simulink library "SG_send_servo_valve_position_command"  (R2025b)
settings: Solver=VariableStepAuto  StartTime=0.0  StopTime=10.0  RelTol=1e-3
libraries: simulink x2, slrealtimeseriallib x2, hdlsllib x1
settings Model: Creator=cmmcguir  LastModifiedBy=cmmcguir

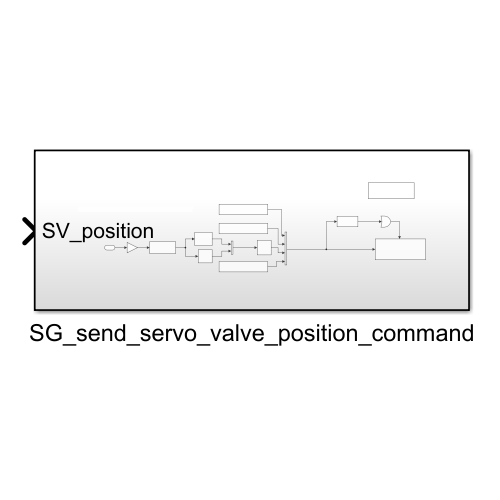
[thumbnail: Simulink's stored preview of the top-level diagram]
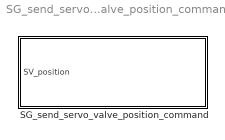
== system SG_send_servo_valve_position_command ==
  SG_send_servo_valve_position_command : Subsystem

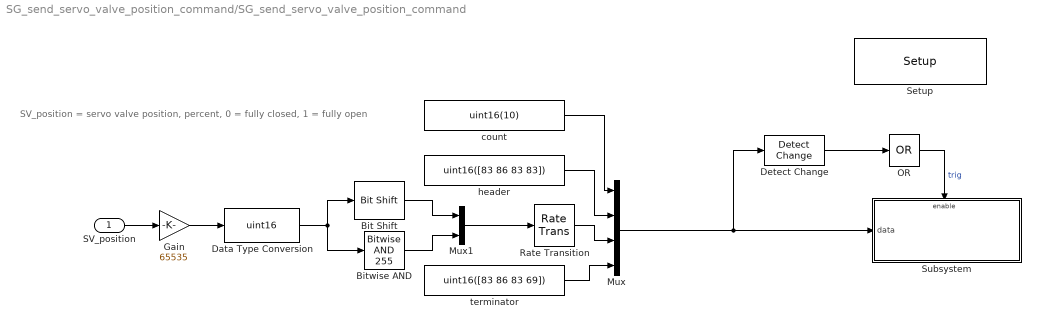
== system SG_send_servo_valve_position_command/SG_send_servo_valve_position_command ==
  note: SV_position = servo valve position, percent, 0 = fully closed, 1 = fully open
  SV_position : Inport
  Bit Shift : hdlsllib/Logic and Bit Operations/Bit Shift  mode=Shift Right Logical  N=8
  Bitwise AND : simulink/Logic and Bit Operations/Bitwise Operator  logicop=AND  UseBitMask=on  BitMask=255  BitMaskRealWorld=Stored Integer
      settings: LibrarySourceBlock=|
      | simulink/Quick Insert/Logic and Bit
      | Operations/Bitwise AND
  Data Type Conversion : DataTypeConversion  OutDataTypeStr=uint16  SaturateOnIntegerOverflow=off  RndMeth=Floor
  Detect Change : simulink/Logic and Bit Operations/Detect Change  vinit=0  OutDataTypeStr=boolean
  Gain : Gain  Gain=65535
  Mux : Mux
  Mux1 : Mux  Inputs=2
  OR : Logic  Operator=OR  Inputs=1  IconShape=distinctive  AllPortsSameDT=off  OutDataTypeStr=boolean
  Rate Transition : RateTransition
  Setup : slrealtimeseriallib/Mainboard/Setup  port=USB Serial Port 1  baud=115200  width=8  nstop=1  parity=None  ctsmode=on
  Subsystem : Subsystem
  count : Constant  Value=uint16(10)
  header : Constant  Value=uint16([83 86 83 83])
  terminator : Constant  Value=uint16([83 86 83 69])
  wires:
  SV_position/1 -> Gain/1
  count/1 -> Mux/1
  Mux1/1 -> Rate Transition/1
  Data Type Conversion/1 -> Bitwise AND/1, Bit Shift/1
  terminator/1 -> Mux/4
  OR/1 -> Subsystem/Enable  "trig"
  Rate Transition/1 -> Mux/3
  Bit Shift/1 -> Mux1/1
  Detect Change/1 -> OR/1
  Bitwise AND/1 -> Mux1/2
  Mux/1 -> Subsystem/1(data), Detect Change/1
  header/1 -> Mux/2
  Gain/1 -> Data Type Conversion/1

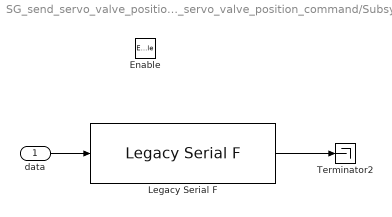
== system SG_send_servo_valve_position_command/SG_send_servo_valve_position_command/Subsystem ==
  data : Inport
  Enable : EnablePort
  Legacy Serial F : slrealtimeseriallib/Mainboard/Legacy Serial F  port=USB Serial Port 1  baud=115200  width=8  nstop=1  parity=None  ctsmode=off  fifosize=1024  idtype=count+16 bit uint  sampletime=.01
  Terminator2 : Terminator
  wires:
  data/1 -> Legacy Serial F/1
  Legacy Serial F/1 -> Terminator2/1
